simulink model "chap1_8"  (Simulink 6.3)
settings: Solver=ode4  StartTime=0.0  StopTime=2  RelTol=1e-3
settings Model: LastModifiedBy=Administrator  ExtModeTrigMode=oneshot  ExtModeArmWhenConnect=off  StrictBusMsg=None
settings DataIOCC: Decimation=100  LimitDataPoints=off  SaveOutput=off  SaveTime=off
settings OptimizationCC: BlockReduction=off  BooleanDataType=off
settings DebuggingCC: SolverPrmCheckMsg=none
settings HardwareCC: TargetUnknown=on

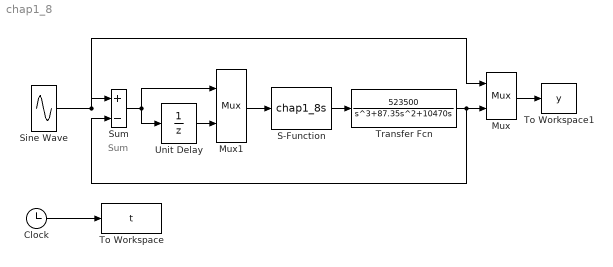
== system chap1_8 ==
  note: Sum
  Clock : Clock
      settings: Decimation=10
  Mux : Mux  Inputs=2
  Mux1 : Mux  Inputs=2
  S-Function : S-Function  FunctionName=chap1_8s
  Sine Wave : Sin  Frequency=1*2*pi  SampleTime=0.001
  Sum : Sum  Inputs=|+-  SaturateOnIntegerOverflow=on  InputSameDT=on
  To Workspace : ToWorkspace  VariableName=t  SampleTime=-1  SaveFormat=Array
  To Workspace1 : ToWorkspace  VariableName=y  SampleTime=-1  SaveFormat=Array
  Transfer Fcn : TransferFcn  Numerator=[523500]  Denominator=[1 87.35 10470 0]
  Unit Delay : UnitDelay  SampleTime=0.001
  wires:
  Sine Wave/1 -> Sum/1, Mux/1
  Mux1/1 -> S-Function/1
  Unit Delay/1 -> Mux1/2
  Sum/1 -> Mux1/1, Unit Delay/1
  S-Function/1 -> Transfer Fcn/1
  Mux/1 -> To Workspace1/1
  Transfer Fcn/1 -> Mux/2, Sum/2
  Clock/1 -> To Workspace/1
